simulink model "IM200HP_Test_Model_v3"  (Simulink 8.1)
settings: Solver=ode45  StartTime=0.0  StopTime=100  RelTol=1e-3
PostLoadFcn:
  | Ts=100e-6;
InitFcn:
  | Ts=100e-6;
undefined symbols (not defined in the file): cb_mech_delay
libraries: powerlib x6, Load_lib x1, Motor_InductionMachine_lib x1, breaker_lib x1
settings Model: Creator=ed12083  LastModifiedBy=ed12083
settings DataIOCC: SignalLoggingSaveFormat=Dataset
settings OptimizationCC: ExpressionDepthLimit=128
settings DebuggingCC: FcnCallInpInsideContextMsg=EnableAllAsError
settings GRTTargetCC: CombineOutputUpdateFcns=on  GRTInterface=off

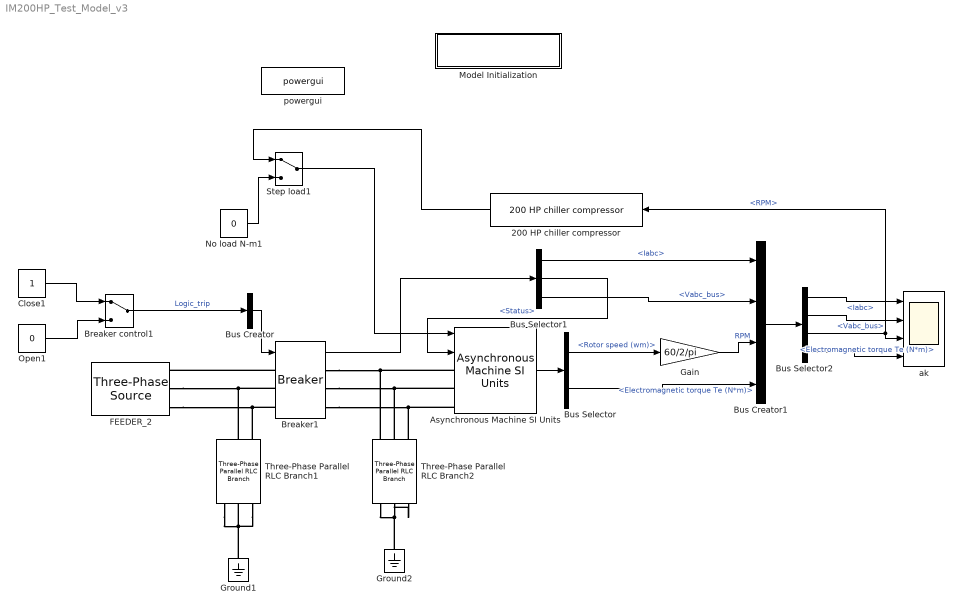
== system IM200HP_Test_Model_v3 ==
  200 HP chiller compressor : Load_lib/200 HP chiller compressor
  Asynchronous Machine SI Units : Motor_InductionMachine_lib/Motor/Asynchronous Machine SI Units  PresetModel=No  MechanicalLoad=Torque Tm  ShowDetailedParameters=on  RotorType=Squirrel-cage  ReferenceFrame=Stationary  NominalParameters=[ 136700/.92/.93, 480, 60 ]  Stator=[ 0.029 0.226/377/1.5]  Rotor=[ 0.022*3 0.226/377/1.5]  Cage1=[ 0.022 0.226/377]  Cage2=[ 0.022 0.226/377]  Lm=13.04/377  Mechanical="[ 63.87 0  2 ]"  PolePairs=2  InitialConditions=[1 0 0 0 0 0 0 0]  Units=SI  LoadFlowParameters=1492000  SimulateSaturation=off  Saturation=[14.03593122, 27.81365428, 53.79336849, 72.68890987, 97.98006896, 148.6815601, 215.7428561, 302.9841135, 420.4778367 ; 230, 322, 414, 460, 506, 552, 598, 644, 690]  TsPowergui=0  TsBlock=-1  IterativeModel=Trapezoidal non iterative  Pmec=0
      settings: AttributesFormatString=\n
  Breaker control1 : ManualSwitch
  Breaker1 : breaker_lib/Breaker  Ts=Ts  mech_delays=[cb_mech_delay(1,:)]
  Bus Creator : BusCreator  Inputs=1
  Bus Creator1 : BusCreator
  Bus Selector : BusSelector  OutputSignals=Mechanical.Rotor speed (wm),Mechanical.Electromagnetic torque Te (N*m)
  Bus Selector1 : BusSelector  OutputSignals=Iabc,Status,Vabc_bus
  Bus Selector2 : BusSelector  OutputSignals=Iabc,Vabc_bus,RPM,Electromagnetic torque Te (N*m)
  Close1 : Constant
  FEEDER_2 : powerlib/Electrical Sources/Three-Phase Source  Voltage=480  PhaseAngle=0  Frequency=60  InternalConnection=Yg  SpecifyImpedance=on  Resistance=0.8929  Inductance=16.58e-3  ShortCircuitLevel=375e6  BaseVoltage=480  XRratio=7.9  BusType=swing  Pref=0  Qref=0  Qmin=-inf  Qmax=inf
  Gain : Gain  Gain=60/2/pi
  Ground1 : powerlib/Elements/Ground  LConnTagsString=a
  Ground2 : powerlib/Elements/Ground  LConnTagsString=a
  Model Initialization : Subsystem  AncestorBlock=artemis/Tools /Misc/Model Initialization  mask(Model Functions){InitFcnX=Ts=100e-6;, prel=off, posl=on, inif=on, strf=off}
      mask prompts: InitFcnX "Initialisation"; prel "Preload Function"; posl "PostLoad Function"; inif "InitFcn"; strf "StartFcn"
      mask init:
      | currentBlock = gcb;
      | root = bdroot(currentBlock);
      | 
      | if ~strcmp(get_param(root,'BlockDiagramType'),'library')
      |     if prel==1
      |         set_param(root, 'PreLoadFcn', InitFcnX);
      |     else
      |         set_param(root, 'PreLoadFcn', '');
      |     end
      |     if inif==1
      |         set_param(root, 'InitFcn', InitFcnX);
      |     else
      |         set_param(root, 'InitFcn', '');
      |     end
      |     if strf==1
      |         set_param(root, 'StartFcn', InitFcnX);
      |     else
      |         set_param(root, 'StartFcn', '');
      |     end
      |     if posl==1
      |         set_param(root, 'PostLoadFcn', InitFcnX);
      |     else
      |         set_param(root, 'PostLoadFcn', '');
      |     end
      | end
      | 
      | pos = get_param(currentBlock, 'Position');
      | width = pos(3) - pos(1); height = pos(4) - pos(2);
      | txt = [ upper(root) '\n' '- InitFcn. . . . . '  get_param(root, 'InitFcn') ];
      settings: CopyFcn=set_param(gcb,'LinkStatus','inactive')
      mask Display: text(5, height*0.5, txt, 'horizontalAlignment', 'left', 'verticalAlignment', 'middle') ;
  No load N-m1 : Constant  Value=0
  Open1 : Constant  Value=0
  Step load1 : ManualSwitch
  Three-Phase Parallel RLC Branch1 : powerlib/Elements/Three-Phase Parallel RLC Branch  LConnTagsString=A|B|C  RConnTagsString=A|B|C  BranchType=R  Resistance=1e6  Inductance=inf  Capacitance=inf  Measurements=None
  Three-Phase Parallel RLC Branch2 : powerlib/Elements/Three-Phase Parallel RLC Branch  LConnTagsString=A|B|C  RConnTagsString=A|B|C  BranchType=RC  Resistance=1e6  Inductance=inf  Capacitance=10e-6  Measurements=None
  ak : Scope  NumInputPorts=4
      settings: ShowLegends=on  YMin=-1750~-450~0~-2000  YMax=1750~450~2000~3500
  powergui : powerlib/powergui  Priority=2  SimulationMode=Discrete  SolverType=Tustin  SampleTime=Ts  frequency=60  SPID=off  DisableSnubberDevices=off  DisableRonSwitches=off  DisableVfSwitches=off  SwTol=0  Interpol=off  DisplayEquations=off  frequencyindice=60  Pbase=100e6  ErrMax=1e-4  Iterations=50  UnitsV=kV  UnitsW=MW  FunctionMessages=off  echomessages=off  HookPort=off  EnableUseOfTLC=off  x0status=blocks  RestoreLinks=warning  ResistiveCurrentMeasurement=off  Frange=logspace(0,3,50)  Ylog=off  Xlog=off  ShowGrid=off  save=off  variable=ZData  structure=0  ZoomFFT=on  StartTime=0.0  cycles=2  DisplayStyle=off  fundamental=60  FreqAxis=off  MaxFrequency=1000  frequencyindicesteady=1  RmsSteady=1  display=off  Ts=0  methode=off
  wires:
  Close1/1 -> Breaker control1/1
  Open1/1 -> Breaker control1/2
  Breaker control1/1 -> Bus Creator/1  "Logic_trip"
  Bus Creator/1 -> Breaker1/1
  Breaker1/1 -> Bus Selector1/1
  Asynchronous Machine SI Units/1 -> Bus Selector/1
  Bus Creator1/1 -> Bus Selector2/1
  Bus Selector2/1 -> ak/1  "<Iabc>"
  Bus Selector2/4 -> ak/4  "<Electromagnetic torque Te (N*m)>"
  Bus Selector2/2 -> ak/2  "<Vabc_bus>"
  Bus Selector1/1 -> Bus Creator1/1  "<Iabc>"
  Bus Selector1/3 -> Bus Creator1/2  "<Vabc_bus>"
  Bus Selector/1 -> Gain/1  "<Rotor speed (wm)>"
  Bus Selector/2 -> Bus Creator1/4  "<Electromagnetic torque Te (N*m)>"
  Gain/1 -> Bus Creator1/3  "RPM"
  Bus Selector2/3 -> ak/3, 200 HP chiller compressor/1  "<RPM>"
  Bus Selector1/2 -> Asynchronous Machine SI Units/2  "<Status>"
  No load N-m1/1 -> Step load1/2
  200 HP chiller compressor/1 -> Step load1/1
  Step load1/1 -> Asynchronous Machine SI Units/1
  connections:
  FEEDER_2/RConn2 -- Breaker1/LConn2 -- Three-Phase Parallel RLC Branch1/RConn2
  FEEDER_2/RConn3 -- Breaker1/LConn3 -- Three-Phase Parallel RLC Branch1/RConn3
  Ground2/LConn1 -- Three-Phase Parallel RLC Branch2/LConn3 -- Three-Phase Parallel RLC Branch2/LConn2 -- Three-Phase Parallel RLC Branch2/LConn1
  Ground1/LConn1 -- Three-Phase Parallel RLC Branch1/LConn3 -- Three-Phase Parallel RLC Branch1/LConn1 -- Three-Phase Parallel RLC Branch1/LConn2
  Three-Phase Parallel RLC Branch2/RConn1 -- Asynchronous Machine SI Units/LConn1 -- Breaker1/RConn1
  Three-Phase Parallel RLC Branch2/RConn2 -- Asynchronous Machine SI Units/LConn2 -- Breaker1/RConn2
  Three-Phase Parallel RLC Branch2/RConn3 -- Breaker1/RConn3 -- Asynchronous Machine SI Units/LConn3
  Breaker1/LConn1 -- FEEDER_2/RConn1

== system IM200HP_Test_Model_v3/Model Initialization ==
